simulink model "RflysimIndoorController_r2018b_V3"  (R2018b)
settings: Solver=ode4  StartTime=0.0  StopTime=inf  FixedStep=ts  MaxStep=0.6  RelTol=1e-3
values from neighbouring files (symbols this model uses):
  l_v = 5    [RflyMain.m]    (also in RflyMain_N12_V6.m; RflyMain_N6_V3.m; RflyMain_N6_V4.m; RflyMain_V2.m)
  p_left_encircle = zeros(length(p_radius(:,1)),2)    [RflyMain.m]
  p_radius = [curve_x;curve_y]'    [RflyMain.m]
  p_right_encircle = zeros(length(p_radius(:,1)),2)    [RflyMain.m]
  p_target = [200,10]    [RflyMain.m]    (also in RflyMain_N12_V6.m; RflyMain_N6_V3.m; RflyMain_N6_V4.m; RflyMain_V2.m)
  ra = 0.6    [RflyMain.m]    (also in RflyMain_N12_V6.m; RflyMain_N6_V3.m; RflyMain_N6_V4.m; RflyMain_V2.m)
  rs = 0.25    [RflyMain.m]    (also in RflyMain_N12_V6.m; RflyMain_N6_V3.m; RflyMain_N6_V4.m; RflyMain_V2.m)
  ts = [0 0]    [QuadModel2D.m]    (also in RflyMain.m = 0.01; RflyMain_N12_V6.m = 0.05; RflyMain_N6_V3.m = 0.05; RflyMain_N6_V4.m = 0.05)
  tunnel_left = [90,20;147,14]    [RflyMain.m]
  tunnel_right = [90,1;147,7]    [RflyMain.m]
  v_max = 2    [RflyMain.m]    (also in RflyMain_N12_V6.m = 3; RflyMain_N6_V3.m = 3; RflyMain_N6_V4.m = 3; RflyMain_V2.m = 3)
undefined symbols (not defined in the file or in its folder): Twist
libraries: robotlib x8, aerolibanimutils x1
settings Model: Creator=51078  LastModifiedBy=51078
settings OptimizationCC: EnhancedBackFolding=on  PassReuseOutputArgsAs=Individual arguments  ZeroExternalMemoryAtStartup=off  ZeroInternalMemoryAtStartup=off  MaxStackSize=64  OptimizeBlockOrder=speed  DifferentSizesBufferReuse=on  OptimizationCustomize=off
settings DebuggingCC: ParameterTunabilityLossMsg=error
settings HardwareCC: ProdBitPerPointer=32  ProdBitPerSizeT=32  ProdBitPerPtrDiffT=32  ProdLargestAtomicFloat=None  ProdIntDivRoundTo=Undefined  ProdEndianess=Unspecified  ProdWordSize=32  ProdHWDeviceType=Generic->Unspecified (assume 32-bit Generic)
settings SFSimCC: SimUseLocalCustomCode=off  MATLABDynamicMemAlloc=off
settings RTWCC: SystemTargetFile=ert.tlc  HardwareBoard=Robot Operating System (ROS)  TLCOptions="-aInlineSetEventsForThisBaseRateFcn=TLC_FALSE -aSuppressMultiTaskScheduler=TLC_FALSE  -aRateBasedStepFcn=0"  TemplateMakefile=ert_default_tmf  RTWUseLocalCustomCode=off  Toolchain=Catkin  TargetLang=C++
settings CodeAppCC: ForceParamTrailComments=on  IgnoreCustomStorageClasses=off  OperatorAnnotations=on  SimulinkDataObjDesc=on  SFDataObjDesc=on  InsertBlockDesc=on

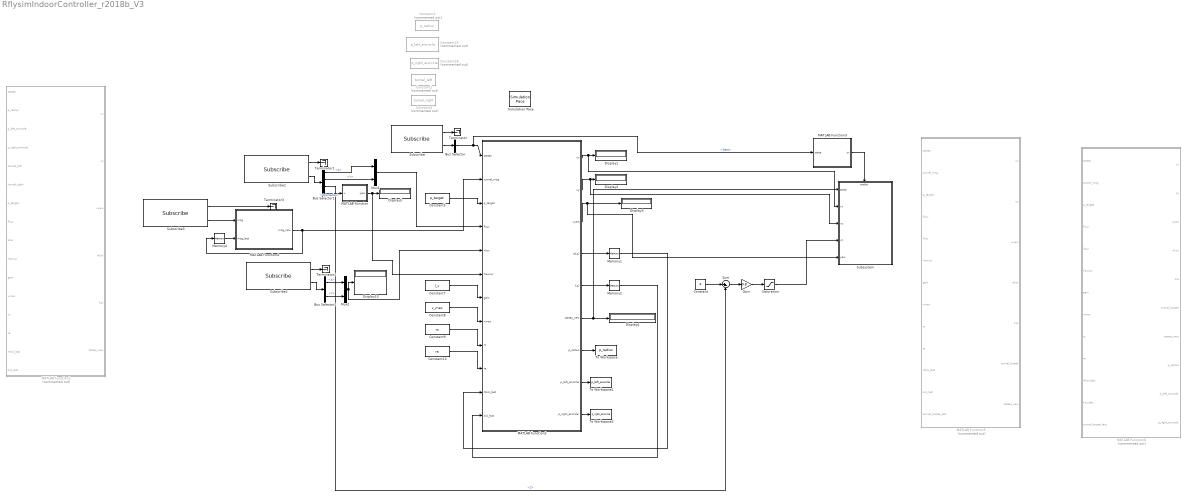
== system RflysimIndoorController_r2018b_V3 ==
  Bus Selector : BusSelector  OutputSignals=Data
  Bus Selector1 : BusSelector  OutputSignals=Pose.Position.X,Pose.Position.Y,Pose.Position.Z,Pose.Orientation
  Bus Selector2 : BusSelector  OutputSignals=Twist.Linear.X,Twist.Linear.Y
  Constant : Constant  Value=4
  Constant1 : Constant  Commented=on  Value=tunnel_left
  Constant10 : Constant  Value=ra
  Constant2 : Constant  Commented=on  Value=p_radius
  Constant25 : Constant  Commented=on  Value=p_left_encircle
  Constant26 : Constant  Commented=on  Value=p_right_encircle
  Constant3 : Constant  Commented=on  Value=tunnel_right
  Constant5 : Constant  Value=p_target
  Constant7 : Constant  Value=l_v
  Constant8 : Constant  Value=v_max
  Constant9 : Constant  Value=rs
  Display{1..5,10} (6 alike) : Display
  Gain : Gain  Gain=0.8
  MATLAB Function : MATLAB Function  TreatAsAtomicUnit=on
  MATLAB Function1 : MATLAB Function  Commented=on  TreatAsAtomicUnit=on
  MATLAB Function2 : MATLAB Function  TreatAsAtomicUnit=on
  MATLAB Function3 : MATLAB Function  TreatAsAtomicUnit=on
  MATLAB Function4 : MATLAB Function  TreatAsAtomicUnit=on
  MATLAB Function5 : MATLAB Function  Commented=on  TreatAsAtomicUnit=on
  MATLAB Function6 : MATLAB Function  Commented=on  TreatAsAtomicUnit=on
  Memory1 : Memory
  Memory2 : Memory
  Memory4 : Memory
  Mux1 : Mux  Inputs=2
  Mux2 : Mux  Inputs=2
  Saturation : Saturate  UpperLimit=2  LowerLimit=-2
  Simulation Pace : aerolibanimutils/Simulation Pace  SimulationPace=1  SleepMode=MATLAB Thread  OutputPaceError=off  SampleTime=ts
  Subscribe : robotlib/Subscribe  topicSource=Select from ROS network  topic=/drone_1/state  messageType=std_msgs/UInt64  sampleTime=-1  messageQueueLength=1
  Subscribe1 : robotlib/Subscribe  topicSource=Select from ROS network  topic=/mavros/local_position/pose  messageType=geometry_msgs/PoseStamped  sampleTime=-1  messageQueueLength=1
  Subscribe2 : robotlib/Subscribe  topicSource=Select from ROS network  topic=/mavros/local_position/velocity_local  messageType=geometry_msgs/TwistStamped  sampleTime=-1  messageQueueLength=1
  Subscribe3 : robotlib/Subscribe  topicSource=Specify your own  topic=/decision_info  messageType=swarm_msgs/Pipeline  sampleTime=-1  messageQueueLength=1
  Subsystem : Subsystem
  Sum : Sum  Inputs=|+-
  Terminator{,1..3} (4 alike) : Terminator
  To Workspace : ToWorkspace  VariableName=p_radius  SaveFormat=Timeseries  SampleTime=-1
  To Workspace1 : ToWorkspace  VariableName=p_left_encircle  SaveFormat=Timeseries  SampleTime=-1
  To Workspace2 : ToWorkspace  VariableName=p_right_encircle  SaveFormat=Timeseries  SampleTime=-1
  wires:
  Subscribe1/1 -> Terminator1/1
  Subscribe1/2 -> Bus Selector1/1
  Bus Selector1/2 -> Mux1/2  "<Y>"
  MATLAB Function2/4(rtksii) -> Memory1/1
  Constant9/1 -> MATLAB Function2/9(rs)
  MATLAB Function2/3(uyaw) -> Subsystem/5(yaw), Display3/1
  Constant5/1 -> MATLAB Function2/3(p_target)
  Constant7/1 -> MATLAB Function2/7(gain)
  Memory1/1 -> MATLAB Function2/11(rtksii_last)
  Constant10/1 -> MATLAB Function2/10(ra)
  Mux2/1 -> MATLAB Function2/5(Vcur), Display10/1
  Memory2/1 -> MATLAB Function2/12(ksii_last)
  Mux1/1 -> MATLAB Function2/4(Pcur)
  MATLAB Function2/1(ux) -> Subsystem/2(vx), Display1/1
  MATLAB Function/1(yaw) -> MATLAB Function2/6(Yawcur), Display5/1
  MATLAB Function2/5(ksii) -> Memory2/1
  Constant8/1 -> MATLAB Function2/8(vmax)
  Subscribe/1 -> Terminator/1
  Subscribe/2 -> Bus Selector/1
  Bus Selector/1 -> MATLAB Function3/1(state), MATLAB Function2/1(states)  "<Data>"
  Bus Selector2/2 -> Mux2/2  "<Y>"
  Bus Selector2/1 -> Mux2/1  "<X>"
  Subscribe2/2 -> Bus Selector2/1
  Subscribe2/1 -> Terminator2/1
  Bus Selector1/4 -> MATLAB Function/1(u)  "<Orientation>"
  MATLAB Function3/1(tri) -> Subsystem/Enable
  MATLAB Function2/6(states_new) -> Subsystem/1(state), Display4/1
  MATLAB Function2/2(uy) -> Subsystem/3(vy), Display2/1
  Bus Selector1/1 -> Mux1/1  "<X>"
  Constant/1 -> Sum/1
  Bus Selector1/3 -> Sum/2  "<Z>"
  Sum/1 -> Gain/1
  Gain/1 -> Saturation/1
  Saturation/1 -> Subsystem/4(vz)
  Subscribe3/1 -> Terminator3/1
  MATLAB Function4/1(msg_new) -> Memory4/1, MATLAB Function2/2(tunnel_msg)
  Subscribe3/2 -> MATLAB Function4/1(msg)
  Memory4/1 -> MATLAB Function4/2(msg_last)
  MATLAB Function2/7(p_radius) -> To Workspace/1
  MATLAB Function2/8(p_left_encircle) -> To Workspace1/1
  MATLAB Function2/9(p_right_encircle) -> To Workspace2/1

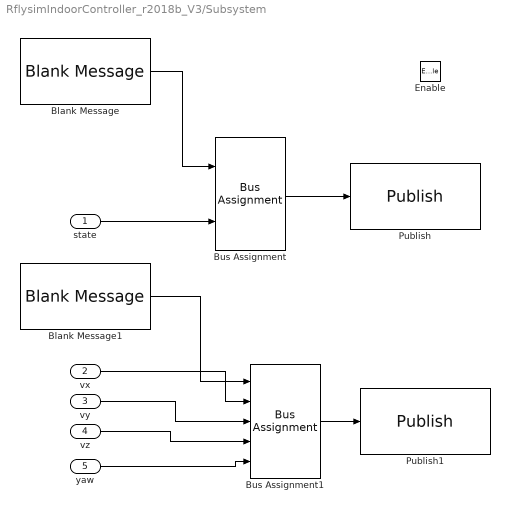
== system RflysimIndoorController_r2018b_V3/Subsystem ==
  state : Inport
  vx : Inport  Port=2
  vy : Inport  Port=3
  vz : Inport  Port=4
  yaw : Inport  Port=5
  Enable : EnablePort
  Blank Message : robotlib/Blank Message  messageClass=Message  entityType=std_msgs/UInt64  messageType=std_msgs/UInt64  SampleTime=inf
  Blank Message1 : robotlib/Blank Message  messageClass=Message  entityType=geometry_msgs/TwistStamped  messageType=geometry_msgs/TwistStamped  SampleTime=inf
  Bus Assignment : BusAssignment  AssignedSignals=Data
  Bus Assignment1 : BusAssignment  AssignedSignals=Twist.Linear.X,Twist.Linear.Y,Twist.Linear.Z,Twist.Angular.Z
  Publish : robotlib/Publish  topicSource=Specify your own  topic=/drone_1/state  messageType=std_msgs/UInt64  messageQueueLength=1
  Publish1 : robotlib/Publish  topicSource=Select from ROS network  topic=/mavros/setpoint_velocity/cmd_vel  messageType=geometry_msgs/TwistStamped  messageQueueLength=1
  wires:
  Blank Message/1 -> Bus Assignment/1
  state/1 -> Bus Assignment/2
  Bus Assignment/1 -> Publish/1
  Bus Assignment1/1 -> Publish1/1
  Blank Message1/1 -> Bus Assignment1/1
  vx/1 -> Bus Assignment1/2
  vy/1 -> Bus Assignment1/3
  yaw/1 -> Bus Assignment1/5
  vz/1 -> Bus Assignment1/4

== matlab function RflysimIndoorController_r2018b_V3/MATLAB Function1 ==
  data: states input; p_radius input; p_left_encircle input; p_right_encircle input; tunnel_left input; ux output; uy output; tunnel_right input; p_target input; Pcur input; Vcur input; Yawcur input; gain input; vmax input; uyaw output; rtksii output size=[N,1]; ksii output size=[N,2]; rs input; ra input; rtksii_last input; ksii_last input; states_new output
function [ux,uy,uyaw,rtksii,ksii,states_new]  = mytunnel(states,p_radius,p_left_encircle,p_right_encircle,tunnel_left,tunnel_right,p_target,Pcur,Vcur,Yawcur,gain,vmax,rs,ra,rtksii_last,ksii_last)
Pcur=Pcur';
Vcur=Vcur';
p_target=p_target';

N=1;
[u_encircle,ux_encircle,uy_encircle,uyaw_encircle,leader_locate,rtksii,ksii,dist_encircle]  = Encirclement(p_radius,p_left_encircle,p_right_encircle,p_target,Pcur,Vcur,Yawcur,gain,vmax,rs,ra,rtksii_last,ksii_last);
[u_pass,ux_pass,uy_pass,tunnel_locate,bottem_tunnel_locate,dist_tunnel]  = TixingTunnel(tunnel_left,tunnel_right,Pcur,Vcur,N,gain,vmax,rs,ra);

ux=zeros(N,1);
uy=zeros(N,1);
uyaw=zeros(N,1);
states_new=0;
if states==20
    ux=ux_encircle;
    uy=uy_encircle;
    uyaw=uyaw_encircle;
    if tunnel_locate~=1
        states_new=20;
    elseif tunnel_locate==1
        states_new=40;
    end
end

if states==40
    ux=ux_pass;
    uy=uy_pass;
    uyaw=zeros(N,1);
    if tunnel_locate==1
        states_new=40;
    elseif tunnel_locate~=1
        states_new=50;
    end
end

== matlab function RflysimIndoorController_r2018b_V3/MATLAB Function2 ==
  data: states input; tunnel_msg input; ux output; uy output; p_target input; Pcur input; Vcur input; Yawcur input; gain input; vmax input; uyaw output; rtksii output size=[N,1]; ksii output size=[N,2]; rs input; ra input; rtksii_last input; ksii_last input; states_new output; p_radius output; p_left_encircle output; p_right_encircle output
function [ux,uy,uyaw,rtksii,ksii,states_new,p_radius,p_left_encircle,p_right_encircle]  = mytunnel(states,tunnel_msg,p_target,Pcur,Vcur,Yawcur,gain,vmax,rs,ra,rtksii_last,ksii_last)
Pcur=Pcur';
Vcur=Vcur';
p_target=p_target';

tunnel_type = tunnel_msg.Pipetype.Data;
point_num=tunnel_msg.Units_SL_Info.CurrentLength;

left_x=zeros(10,1);
left_y=zeros(10,1);
right_x=zeros(10,1);
right_y=zeros(10,1);
middle_x=zeros(10,1);
middle_y=zeros(10,1);


for i=1:point_num
    left_x(i,1) = tunnel_msg.Units(i).Left.X;
    left_y(i,1) = tunnel_msg.Units(i).Left.Y;
    
    right_x(i,1) = tunnel_msg.Units(i).Right.X;
    right_y(i,1) = tunnel_msg.Units(i).Right.Y;
    
    middle_x(i,1) = tunnel_msg.Units(i).Middle.X;
    middle_y(i,1) = tunnel_msg.Units(i).Middle.Y;
end

left_x=left_x(1:point_num,1);
left_y=left_y(1:point_num,1);
right_x=right_x(1:point_num,1);
right_y=right_y(1:point_num,1);
middle_x=middle_x(1:point_num,1);
middle_y=middle_y(1:point_num,1);



inter_num = 100;
p_radius=zeros(inter_num,2);
p_left_encircle=zeros(inter_num,2);
p_right_encircle=zeros(inter_num,2);

if tunnel_type==10
    k=1:length(middle_x);
    ki=linspace(1,length(middle_x),inter_num); %%%%% 插值的点越多，控制更精确，曲线更光滑，计算更耗时
    p_radius_x=(interp1(k,middle_x,ki,'pchip'))';
    p_radius_y=(interp1(k,middle_y,ki,'pchip'))';
    for i=1:length(p_radius(:,1))
        p_radius(i,1)=p_radius_x(i);
        p_radius(i,2)=p_radius_y(i);
    end
    
    k=1:length(left_x);
    ki=linspace(1,length(left_x),inter_num); %%%%% 插值的点越多，控制更精确，曲线更光滑，计算更耗时
    p_left_encircle_x=(interp1(k,left_x,ki,'pchip'))';
    p_left_encircle_y=(interp1(k,left_y,ki,'pchip'))';
    for i=1:length(p_left_encircle(:,1))
        p_left_encircle(i,1)=p_left_encircle_x(i);
        p_left_encircle(i,2)=p_left_encircle_y(i);
    end
    
    k=1:length(right_x);
    ki=linspace(1,length(right_x),inter_num); %%%%% 插值的点越多，控制更精确，曲线更光滑，计算更耗时
    p_right_encircle_x=(interp1(k,right_x,ki,'pchip'))';
    p_right_encircle_y=(interp1(k,right_y,ki,'pchip'))';
    for i=1:length(p_right_encircle(:,1))
        p_right_encircle(i,1)=p_right_encircle_x(i);
        p_right_encircle(i,2)=p_right_encircle_y(i);
    end
end


N=1;

ux=zeros(N,1);
uy=zeros(N,1);
uyaw=zeros(N,1);
states_new=0;

[u_encircle,ux_encircle,uy_encircle,uyaw_encircle,leader_locate,rtksii,ksii,dist_encircle]  = Encirclement(p_radius,p_left_encircle,p_right_encircle,p_target,Pcur,Vcur,Yawcur,gain,vmax,rs,ra,rtksii_last,ksii_last);


if states==30
    states_new=30;
    ux=ux_encircle;
    uy=uy_encircle;
    uyaw=uyaw_encircle;
    if abs(leader_locate-inter_num)<5
        states_new=20;
    end
end

== matlab function RflysimIndoorController_r2018b_V3/MATLAB Function ==
  data: u input; yaw output
function yaw = fcn(u)
q0=u.W;
q1=u.X;
q2=u.Y;
q3=u.Z;
yaw = atan2(2*(q0*q3+q1*q2), 1-2*(q2*q2+q3*q3));

== matlab function RflysimIndoorController_r2018b_V3/MATLAB Function3 ==
  data: state input; tri output
function tri = fcn(state)
tri=0;
if state==30 
    tri=1;
end

== matlab function RflysimIndoorController_r2018b_V3/MATLAB Function4 ==
  data: msg input; msg_new output Bus: SL_Bus_RflysimIndoorController_r_Pipeline_8k4wqz; msg_last input
function msg_new = fcn(msg,msg_last)
if msg.Units_SL_Info.CurrentLength==0
    msg_new=msg_last;
else
    msg_new=msg;
end

== matlab function RflysimIndoorController_r2018b_V3/MATLAB Function5 ==
  data: states input; tunnel_msg input; ux output; uy output; p_target input; Pcur input; Vcur input; Yawcur input; gain input; vmax input; uyaw output; rtksii output size=[N,1]; ksii output size=[N,2]; tunnel_locate output; rs input; ra input; rtksii_last input; ksii_last input; states_new output; tunnel_locate_last input
function [ux,uy,uyaw,rtksii,ksii,tunnel_locate,states_new]  = mytunnel(states,tunnel_msg,p_target,Pcur,Vcur,Yawcur,gain,vmax,rs,ra,rtksii_last,ksii_last,tunnel_locate_last)
Pcur=Pcur';
Vcur=Vcur';
p_target=p_target';

tunnel_type = tunnel_msg.Pipetype.Data;
% point_num=tunnel_msg.Units_SL_Info.CurrentLength;
point_num=3;

left_x=zeros(point_num,1);
left_y=zeros(point_num,1);
right_x=zeros(point_num,1);
right_y=zeros(point_num,1);
middle_x=zeros(point_num,1);
middle_y=zeros(point_num,1);

for i=1:point_num
    if tunnel_type==10 %%曲线管道
        left_x(i,1) = tunnel_msg.Units(i).Left.X;
        left_y(i,1) = tunnel_msg.Units(i).Left.Y;
        
        right_x(i,1) = tunnel_msg.Units(i).Right.X;
        right_y(i,1) = tunnel_msg.Units(i).Right.Y;
        
        middle_x(i,1) = tunnel_msg.Units(i).Middle.X;
        middle_y(i,1) = tunnel_msg.Units(i).Middle.Y;
    elseif tunnel_type==20 %%梯形管道
        left_x(i,1) = tunnel_msg.Units(i).Left.X;
        left_y(i,1) = tunnel_msg.Units(i).Left.Y;
        
        right_x(i,1) = tunnel_msg.Units(i).Right.X;
        right_y(i,1) = tunnel_msg.Units(i).Right.Y;
    end
end

inter_num = 100;
p_radius=zeros(inter_num,2);
p_left_encircle=zeros(inter_num,2);
p_right_encircle=zeros(inter_num,2);
tunnel_left=zeros(point_num,2);
tunnel_right=zeros(point_num,2);

if tunnel_type==10
    
    k=1:length(middle_x);
    ki=linspace(1,length(middle_x),inter_num); %%%%% 插值的点越多，控制更精确，曲线更光滑，计算更耗时
    p_radius_x=(interp1(k,middle_x,ki,'pchip'))';
    p_radius_y=(interp1(k,middle_y,ki,'pchip'))';
    for i=1:length(p_radius(:,1))
        p_radius(i,1)=p_radius_x(i);
        p_radius(i,2)=p_radius_y(i);
    end
    
    k=1:length(left_x);
    ki=linspace(1,length(left_x),inter_num); %%%%% 插值的点越多，控制更精确，曲线更光滑，计算更耗时
    p_left_encircle_x=(interp1(k,left_x,ki,'pchip'))';
    p_left_encircle_y=(interp1(k,left_y,ki,'pchip'))';
    for i=1:length(p_left_encircle(:,1))
        p_left_encircle(i,1)=p_left_encircle_x(i);
        p_left_encircle(i,2)=p_left_encircle_y(i);
    end
    
    k=1:length(right_x);
    ki=linspace(1,length(right_x),inter_num); %%%%% 插值的点越多，控制更精确，曲线更光滑，计算更耗时
    p_right_encircle_x=(interp1(k,right_x,ki,'pchip'))';
    p_right_encircle_y=(interp1(k,right_y,ki,'pchip'))';
    for i=1:length(p_right_encircle(:,1))
        p_right_encircle(i,1)=p_right_encircle_x(i);
        p_right_encircle(i,2)=p_right_encircle_y(i);
    end
elseif tunnel_type==20
    tunnel_left=[left_x,left_y];
    tunnel_right=[right_x,right_y];
end

N=1;
[u_encircle,ux_encircle,uy_encircle,uyaw_encircle,leader_locate,rtksii,ksii,dist_encircle]  = Encirclement(p_radius,p_left_encircle,p_right_encircle,p_target,Pcur,Vcur,Yawcur,gain,vmax,rs,ra,rtksii_last,ksii_last);
[u_pass,ux_pass,uy_pass,tunnel_locate,bottem_tunnel_locate,dist_tunnel]  = TixingTunnel(tunnel_left,tunnel_right,Pcur,Vcur,N,gain,vmax,rs,ra);

ux=zeros(N,1);
uy=zeros(N,1);
uyaw=zeros(N,1);
states_new=0;
% if states==30
%     if tunnel_locate==0 && tunnel_locate_last <= tunnel_locate
%         ux=ux_encircle;
%         uy=uy_encircle;
%         uyaw=uyaw_encircle;
%         if abs(leader_locate-inter_num)<5
%             states_new=20;
%         end
%     elseif tunnel_locate~=0
%         ux=ux_pass;
%         uy=uy_pass;
%     elseif tunnel_locate==0 && tunnel_locate_last > tunnel_locate
%         states_new=20;
%     end
% end
if states==30
    states_new=30;
    if tunnel_type==10
        ux=ux_encircle;
        uy=uy_encircle;
        uyaw=uyaw_encircle;
        if abs(leader_locate-inter_num)<5
            states_new=20;
        end
    elseif tunnel_type==20
        ux=ux_pass;
        uy=uy_pass;
        if tunnel_locate==0 && tunnel_locate_last > tunnel_locate
            states_new=20;
        end
    end
end

== matlab function RflysimIndoorController_r2018b_V3/MATLAB Function6 ==
  data: states input; tunnel_msg input; ux output; uy output; p_target input; Pcur input; Vcur input; Yawcur input; gain input; vmax input; uyaw output; rtksii output size=[N,1]; ksii output size=[N,2]; tunnel_locate output; rs input; ra input; rtksii_last input; ksii_last input; states_new output; tunnel_locate_last input; p_radius output; p_left_encircle output; p_right_encircle output
function [ux,uy,uyaw,rtksii,ksii,tunnel_locate,states_new,p_radius,p_left_encircle,p_right_encircle]  = mytunnel(states,tunnel_msg,p_target,Pcur,Vcur,Yawcur,gain,vmax,rs,ra,rtksii_last,ksii_last,tunnel_locate_last)
Pcur=Pcur';
Vcur=Vcur';
p_target=p_target';

tunnel_type = tunnel_msg.Pipetype.Data;
point_num=tunnel_msg.Units_SL_Info.CurrentLength;

left_x=zeros(10,1);
left_y=zeros(10,1);
right_x=zeros(10,1);
right_y=zeros(10,1);
middle_x=zeros(10,1);
middle_y=zeros(10,1);
tunnel_left=zeros(10,2);
tunnel_right=zeros(10,2);

for i=1:point_num
    left_x(i,1) = tunnel_msg.Units(i).Left.X;
    left_y(i,1) = tunnel_msg.Units(i).Left.Y;
    
    right_x(i,1) = tunnel_msg.Units(i).Right.X;
    right_y(i,1) = tunnel_msg.Units(i).Right.Y;
    
    middle_x(i,1) = tunnel_msg.Units(i).Middle.X;
    middle_y(i,1) = tunnel_msg.Units(i).Middle.Y;
end

left_x=left_x(1:point_num,1);
left_y=left_y(1:point_num,1);
right_x=right_x(1:point_num,1);
right_y=right_y(1:point_num,1);
middle_x=middle_x(1:point_num,1);
middle_y=middle_y(1:point_num,1);



inter_num = 100;
p_radius=zeros(inter_num,2);
p_left_encircle=zeros(inter_num,2);
p_right_encircle=zeros(inter_num,2);
if tunnel_type==10
    k=1:length(middle_x);
    ki=linspace(1,length(middle_x),inter_num); %%%%% 插值的点越多，控制更精确，曲线更光滑，计算更耗时
    p_radius_x=(interp1(k,middle_x,ki,'pchip'))';
    p_radius_y=(interp1(k,middle_y,ki,'pchip'))';
    for i=1:length(p_radius(:,1))
        p_radius(i,1)=p_radius_x(i);
        p_radius(i,2)=p_radius_y(i);
    end
    
    k=1:length(left_x);
    ki=linspace(1,length(left_x),inter_num); %%%%% 插值的点越多，控制更精确，曲线更光滑，计算更耗时
    p_left_encircle_x=(interp1(k,left_x,ki,'pchip'))';
    p_left_encircle_y=(interp1(k,left_y,ki,'pchip'))';
    for i=1:length(p_left_encircle(:,1))
        p_left_encircle(i,1)=p_left_encircle_x(i);
        p_left_encircle(i,2)=p_left_encircle_y(i);
    end
    
    k=1:length(right_x);
    ki=linspace(1,length(right_x),inter_num); %%%%% 插值的点越多，控制更精确，曲线更光滑，计算更耗时
    p_right_encircle_x=(interp1(k,right_x,ki,'pchip'))';
    p_right_encircle_y=(interp1(k,right_y,ki,'pchip'))';
    for i=1:length(p_right_encircle(:,1))
        p_right_encircle(i,1)=p_right_encircle_x(i);
        p_right_encircle(i,2)=p_right_encircle_y(i);
    end
elseif tunnel_type==20
    tunnel_left=[left_x,left_y];
    tunnel_right=[right_x,right_y];
end


N=1;

ux=zeros(N,1);
uy=zeros(N,1);
uyaw=zeros(N,1);
states_new=0;
tunnel_locate=0;
ux_pass=0;
uy_pass=0;
    
[u_encircle,ux_encircle,uy_encircle,uyaw_encircle,leader_locate,rtksii,ksii,dist_encircle]  = Encirclement(p_radius,p_left_encircle,p_right_encircle,p_target,Pcur,Vcur,Yawcur,gain,vmax,rs,ra,rtksii_last,ksii_last);
if sum(sum(tunnel_left))~=0
    [u_pass,ux_pass,uy_pass,tunnel_locate,bottem_tunnel_locate,dist_tunnel]  = TixingTunnel(tunnel_left,tunnel_right,Pcur,Vcur,N,gain,vmax,rs,ra);
end

if states==30
    states_new=30;
    if tunnel_type==10
        ux=ux_encircle;
        uy=uy_encircle;
        uyaw=uyaw_encircle;
        if abs(leader_locate-inter_num)<5
            states_new=20;
        end
    elseif tunnel_type==20
        ux=ux_pass;
        uy=uy_pass;
        if tunnel_locate==0 && tunnel_locate_last > tunnel_locate
            states_new=20;
        end
    end
end
